simulink model "Predefined_with_GroundTruth_mod22vig1"  (R2022b)
settings: Solver=ode45  StartTime=0.0  StopTime=inf  MaxStep=0.01  RelTol=1e-3
PreLoadFcn:
  | old_index = 1;
model workspace (MAT data in the model file):
  firstWarning = 1
  originalScenarioChecksum = '114339432DE22364D47BB28FC96DC10C'
undefined symbols (not defined in the file or in its folder): Acceleration, ActorID, AngularVelocity, curvature, curvatureAhd, DefaultGear, DEND_B, DEND_S, DEND_T, direction, DiscIntNeverNeededParam, driving, gradbp, L, LF, LR, matlabshared, MAX_BRAKE, MAX_STEER, MAX_TORQUE, MCAR, MIN_BRAKE, MIN_STEER, MIN_TORQUE, NUMD_B, NUMD_S, NUMD_T, Pitch, Position, psi_o, R, Roll, RRdamp, SceneInfo, session, sigbuilder_block, STEER_RATIO, stopSign_ID, Tdead, thetaRefs, TL_ID, TrackWidth, Ts, ts, Vdead, Velocity, WB, X_o, xRef2, xRef2s, Y_o, Yaw, yRef2, yRef2s
libraries: mpcsigdimcheck_private x10, drivingscenarioandsensors x8, drivingvehiclecontroller x2, eeGeneralControl x2, slpidlib x2, simulink x2, trackingutilitieslib x2, mpclib x1, mpcadaslib x1, robotalgslib x1, simulink_extras x1, drivinglib x1
(part 2 of 3)

== system Predefined_with_GroundTruth_mod22vig1/Subsystem/Tracking ==
  Detections : Inport
  Camera : drivingscenarioandsensors/Vision Detection Generator  SensorIndex=1  DetectorOutput=Objects only  UpdateInterval=0.01  LaneUpdateInterval=0.1  SensorLocation=[1.9 0]  Height=1.1  Yaw=0  Pitch=1  Roll=0  BusNameSource=Auto  BusName=BusObjectDetections  BusName2Source=Auto  BusName2=BusLaneDetections  MaxNumDetectionsSource=Property  MaxNumDetections=10  MaxNumLanesSource=Property  MaxNumLanes=30  DetectionCoordinates=Ego Cartesian  SimulateUsing=Interpreted execution  MaxRange=150  BoundingBoxAccuracy=5  ProcessNoiseIntensity=5  MaxSpeed=100  MaxAllowedOcclusion=0.5  MinObjectImageSize=[2 2]  DetectionProbability=0.9  FalsePositivesPerImage=0.1  MinLaneImageSize=[20 3]  LaneBoundaryAccuracy=3  HasNoise=on  InitialSeedSource=Repeatable  InitialSeed=0  UsedSeed=0  ActorProfilesSource=From Scenario Reader block  ActorProfilesParameters=driving.internal.ActorProfilesParameters  ActorProfilesExpression=[struct('ActorID',1,'ClassID',1,'Length',4.7,'Width',1.8,'Height',1.4,'OriginOffset',[-1.35 0 0],'MeshVertices',[3.7 0.9 0.857439446366782;3.7 -0.9 0.857439446366782;3.7 -0.9 0.314878892733564;3.7 0.9 0.314878892733564;3.7 0.9 0.857439446366782;2.525 0.9 0.993079584775086;2.525 -0.9 0.993079584775086;3.7 -0.9 0.857439446366782;1.82 0.72 1.4;0.41 0.72 1.4;0.41 -0.72 1.4;1.82 -0.72 1.4;-0.295 0.9 0.993079584775086;-1 0.9 0.857439446366782;-1 -0.9 0.857439446366782;-0.295 -0.9 0.993079584775086;3.7 0.9 0.857439446366782;3.7 0.9 0.314878892733564;2.525 0.9 0.314878892733564;2.525 0.9 0.993079584775086;2.525 0.9 0.993079584775086;2.525 0.9 0.314878892733564;-0.295 0.9 0.314878892733564;-0.295 0.9 0.993079584775086;-0.295 0.9 0.993079584775086;-0.295 0.9 0.314878892733564;-1 0.9 0.355570934256055;-1 0.9 0.857439446366782;2.525 0.9 0.993079584775086;-0.295 0.9 0.993079584775086;0.41 0.72 1.4;1.82 0.72 1.4;3.7 -0.9 0.857439446366782;3.7 -0.9 0.314878892733564;2.525 -0.9 0.314878892733564;2.525 -0.9 0.993079584775086;2.525 -0.9 0.993079584775086;2.525 -0.9 0.314878892733564;-0.295 -0.9 0.314878892733564;-0.295 -0.9 0.993079584775086;-0.295 -0.9 0.993079584775086;-0.295 -0.9 0.314878892733564;-1 -0.9 0.355570934256055;-1 -0.9 0.857439446366782;2.525 -0.9 0.993079584775086;-0.295 -0.9 0.993079584775086;0.41 -0.72 1.4;1.82 -0.72 1.4;-0.295 0.9 0.993079584775086;-0.295 -0.9 0.993079584775086;0.41 -0.72 1.4;0.41 0.72 1.4;2.525 -0.9 0.993079584775086;1.82 -0.72 1.4;1.82 0.72 1.4;2.525 0.9 0.993079584775086;-1 0.9 0.857439446366782;-1 0.9 0.355570934256055;-1 -0.9 0.355570934256055;-1 -0.9 0.857439446366782;3.7 0.9 0.314878892733564;3.7 -0.9 0.314878892733564;-0.295 -0.9 0.314878892733564;-0.295 0.9 0.314878892733564;-0.295 0.9 0.314878892733564;-1 0.9 0.355570934256055;-1 -0.9 0.355570934256055;-0.295 -0.9 0.314878892733564;0 -0.63 0;0 -0.87 0;0.191030206995054 -0.63 0.0601365173421445;0.191030206995054 -0.87 0.0601365173421445;0.309093367795925 -0.63 0.217575963708927;0.309093367795925 -0.87 0.217575963708927;0.309093367795925 -0.63 0.412181821758201;0.309093367795925 -0.87 0.412181821758201;0.191030206995054 -0.63 0.569621268124983;0.191030206995054 -0.87 0.569621268124983;0 -0.63 0.629757785467128;0 -0.87 0.629757785467128;-0.191030206995054 -0.63 0.569621268124983;-0.191030206995054 -0.87 0.569621268124983;-0.309093367795925 -0.63 0.412181821758201;-0.309093367795925 -0.87 0.412181821758201;-0.309093367795925 -0.63 0.217575963708927;-0.309093367795925 -0.87 0.217575963708927;-0.191030206995054 -0.63 0.0601365173421445;-0.191030206995054 -0.87 0.0601365173421445;0 -0.63 0;0 -0.87 0;0 -0.63 0;0.191030206995054 -0.63 0.0601365173421445;0.309093367795925 -0.63 0.217575963708927;0.309093367795925 -0.63 0.412181821758201;0.191030206995054 -0.63 0.569621268124983;0 -0.63 0.629757785467128;-0.191030206995054 -0.63 0.569621268124983;-0.309093367795925 -0.63 0.412181821758201;-0.309093367795925 -0.63 0.217575963708927;-0.191030206995054 -0.63 0.0601365173421445;0 -0.87 0;0.191030206995054 -0.87 0.0601365173421445;0.309093367795925 -0.87 0.217575963708927;0.309093367795925 -0.87 0.412181821758201;0.191030206995054 -0.87 0.569621268124983;0 -0.87 0.629757785467128;-0.191030206995054 -0.87 0.569621268124983;-0.309093367795925 -0.87 0.412181821758201;-0.309093367795925 -0.87 0.217575963708927;-0.191030206995054 -0.87 0.0601365173421445;0 0.87 0;0 0.63 0;0.191030206995054 0.87 0.0601365173421445;0.191030206995054 0.63 0.0601365173421445;0.309093367795925 0.87 0.217575963708927;0.309093367795925 0.63 0.217575963708927;0.309093367795925 0.87 0.412181821758201;0.309093367795925 0.63 0.412181821758201;0.191030206995054 0.87 0.569621268124983;0.191030206995054 0.63 0.569621268124983;0 0.87 0.629757785467128;0 0.63 0.629757785467128;-0.191030206995054 0.87 0.569621268124983;-0.191030206995054 0.63 0.569621268124983;-0.309093367795925 0.87 0.412181821758201;-0.309093367795925 0.63 0.412181821758201;-0.309093367795925 0.87 0.217575963708927;-0.309093367795925 0.63 0.217575963708927;-0.191030206995054 0.87 0.0601365173421445;-0.191030206995054 0.63 0.0601365173421445;0 ...(+3718 chars)],'MeshFaces',[1 2 3;3 4 1;5 6 7;7 8 5;9 10 11;11 12 9;13 14 15;15 16 13;17 18 19;19 20 17;21 22 23;23 24 21;25 26 27;27 28 25;29 30 31;31 32 29;33 34 35;35 36 33;37 38 39;39 40 37;41 42 43;43 44 41;45 46 47;47 48 45;49 50 51;51 52 49;53 54 55;55 56 53;57 58 59;59 60 57;61 62 63;63 64 61;65 66 67;67 68 65;69 71 72;72 70 69;71 73 74;74 72 71;73 75 76;76 74 73;75 77 78;78 76 75;77 79 80;80 78 77;79 81 82;82 80 79;81 83 84;84 82 81;83 85 86;86 84 83;85 87 88;88 86 85;87 89 90;90 88 87;91 92 93;91 93 94;91 94 95;91 95 96;91 96 97;91 97 98;91 98 99;91 99 100;101 102 103;101 103 104;101 104 105;101 105 106;101 106 107;101 107 108;101 108 109;101 109 110;111 113 114;114 112 111;113 115 116;116 114 113;115 117 118;118 116 115;117 119 120;120 118 117;119 121 122;122 120 119;121 123 124;124 122 121;123 125 126;126 124 123;125 127 128;128 126 125;127 129 130;130 128 127;129 131 132;132 130 129;133 134 135;133 135 136;133 136 137;133 137 138;133 138 139;133 139 140;133 140 141;133 141 142;143 144 145;143 145 146;143 146 147;143 147 148;143 148 149;143 149 150;143 150 151;143 151 152;153 155 156;156 154 153;155 157 158;158 156 155;157 159 160;160 158 157;159 161 162;162 160 159;161 163 164;164 162 161;163 165 166;166 164 163;165 167 168;168 166 165;167 169 170;170 168 167;169 171 172;172 170 169;171 173 174;174 172 171;175 176 177;175 177 178;175 178 179;175 179 180;175 180 181;175 181 182;175 182 183;175 183 184;185 186 187;185 187 188;185 188 189;185 189 190;185 190 191;185 191 192;185 192 193;185 193 194;195 197 198;198 196 195;197 199 200;200 198 197;199 201 202;202 200 199;201 203 204;204 202 201;203 205 206;206 204 203;205 207 208;208 206 205;207 209 210;210 208 207;209 211 212;212 210 209;211 213 214;214 212 211;213 215 216;216 214 213;217 218 219;217 219 220;217 220 221;217 221 222;217 222 223;217 223 224;217 224 225;217 225 226;227 228 229;227 229 230;227 230 231;227 231 232;227 232 233;227 233 234;227 234 235;227 235 236],'RCSPattern',[10 10;10 10],'RCSAzimuthAngles',[-180 180],'RCSElevationAngles',[-90 90]); struct('ActorID',2,'ClassID',7,'Length',0.7,'Width',0.2,'Height',0.1,'OriginOffset',[0 0 0],'MeshVertices',[0.35 -0.1 0.1;0.35 0.1 0.1;-0.35 0.1 0.1;-0.35 -0.1 0.1;0.35 -0.1 0;0.35 0.1 0;-0.35 0.1 0;-0.35 -0.1 0],'MeshFaces',[6 2 1;1 5 6;8 4 3;3 7 8;6 7 3;3 2 6;5 1 4;4 8 5;4 1 2;2 3 4;7 6 5;5 8 7],'RCSPattern',[10 10;10 10],'RCSAzimuthAngles',[-180 180],'RCSElevationAngles',[-90 90])]  Intrinsics=driving.internal.cameraIntrinsics('FocalLength',[400 800],'PrincipalPoint',[320 240],'ImageSize',[480 640],'RadialDistortion',[0 0],'TangentialDistortion',[0 0],'Skew',0)
  Detection Concatenation : trackingutilitieslib/Detection Concatenation  NumInputs=2  BusNameSource=Property  BusName=Detections  SimulateUsing=Interpreted execution
  Multi-Object Tracker : drivinglib/Multi-Object Tracker  TrackerIndex=uint32( 0 )  FilterInitializationFcn=helperInitSimulinkDemoFilter  AssignmentThreshold=50  ConfirmationThreshold=[ 2, 3 ]  DeletionThreshold=[ 5, 5 ]  MaxNumTracks=20  MaxNumSensors=20  OOSMHandling=Neglect  StateParametersSimulink=struct  HasStateParametersInput=off  TimeInputSource=Auto  HasCostMatrixInput=off  HasDetectableTrackIDsInput=off  BusNameSource=Auto  BusName=BusMultiObjectTracker  TentativeTracksOutputPort=off  AllTracksOutputPort=off  SimulateUsing=Interpreted execution
  Radar Detection Generator : drivingscenarioandsensors/Radar Detection Generator  SensorIndex=2  UpdateInterval=0.01  SensorLocation=[ 1.5, 0 ]  Height=0.2  Yaw=0  Pitch=0  Roll=0  BusNameSource=Auto  BusName=BusRadarDetectionGenerator  MaxNumDetectionsSource=Property  MaxNumDetections=50  DetectionCoordinates=Ego Cartesian  SimulateUsing=Interpreted execution  AzimuthResolution=4  ElevationResolution=10  RangeResolution=2.5  RangeRateResolution=0.5  AzimuthBiasFraction=0.1  ElevationBiasFraction=0.1  RangeBiasFraction=0.05  RangeRateBiasFraction=0.05  FieldOfView=[ 60, 5 ]  MaxRange=150  RangeRateLimits=[ -100, 100 ]  DetectionProbability=0.9  FalseAlarmRate=1e-6  ReferenceRange=100  ReferenceRCS=0  HasElevation=off  HasRangeRate=on  HasNoise=on  HasFalseAlarms=on  HasOcclusion=on  InitialSeedSource=Repeatable  InitialSeed=0  UsedSeed=matlabshared.tracking.internal.SimulinkUtilities.seedManager(gcb)  ActorProfilesSource=Parameters  ActorProfilesParameters=driving.internal.ActorProfilesRadarParameters  ActorProfilesExpression=struct( 'ClassID', 0, 'Length', 4.7, 'Width', 1.8, 'Height', 1.4, 'OriginOffset', [ -1.35, 0, 0 ], 'RCSPattern', [ 10, 10; 10, 10 ], 'RCSAzimuthAngles', [ -180, 180 ], 'RCSElevationAngles', [ -90, 90 ] )
  Subsystem1 : Subsystem  Commented=on
  Confirmed_Tracks : Outport
  wires:
  Camera/1 -> Detection Concatenation/1  "Camera Detections"
  Radar Detection Generator/1 -> Detection Concatenation/2  "Lidar Detections"
  Detections/1 -> Radar Detection Generator/1, Camera/1
  Detection Concatenation/1 -> Multi-Object Tracker/1
  Multi-Object Tracker/1 -> Confirmed_Tracks/1

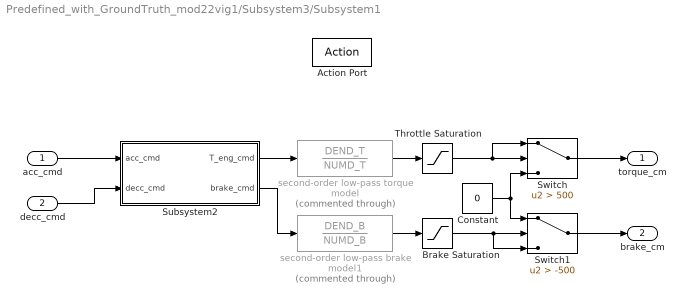
== system Predefined_with_GroundTruth_mod22vig1/Subsystem3/Subsystem1 ==
  acc_cmd : Inport
  decc_cmd : Inport  Port=2
  Action Port : ActionPort  ActionPortLabel=case [ 0 ]:
  Brake Saturation : Saturate  UpperLimit=MAX_BRAKE  LowerLimit=MIN_BRAKE
  Constant : Constant  Value=0
  Subsystem2 : Subsystem
  Switch : Switch  Criteria=u2 > Threshold  Threshold=500  SaturateOnIntegerOverflow=off  InputSameDT=off
  Switch1 : Switch  Criteria=u2 > Threshold  Threshold=-500  SaturateOnIntegerOverflow=off  InputSameDT=off
  Throttle Saturation : Saturate  UpperLimit=MAX_TORQUE  LowerLimit=MIN_TORQUE
  second-order low-pass brake model1 : DiscreteTransferFcn  Commented=through  Numerator=DEND_B  Denominator=NUMD_B  SampleTime=ts
  second-order low-pass torque model : DiscreteTransferFcn  Commented=through  Numerator=DEND_T  Denominator=NUMD_T  SampleTime=ts
  torque_cm : Outport
  brake_cm : Outport  Port=2
  wires:
  Subsystem2/1(T_eng_cmd) -> second-order low-pass torque model/1
  acc_cmd/1 -> Subsystem2/1(acc_cmd)
  second-order low-pass brake model1/1 -> Brake Saturation/1
  Subsystem2/2(brake_cmd) -> second-order low-pass brake model1/1
  decc_cmd/1 -> Subsystem2/2(decc_cmd)
  second-order low-pass torque model/1 -> Throttle Saturation/1
  Throttle Saturation/1 -> Switch/2, Switch/1
  Switch/1 -> torque_cm/1
  Brake Saturation/1 -> Switch1/2, Switch1/3
  Switch1/1 -> brake_cm/1
  Constant/1 -> Switch/3, Switch1/1

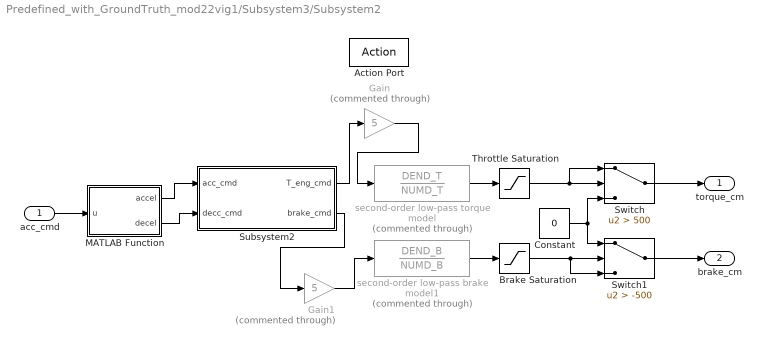
== system Predefined_with_GroundTruth_mod22vig1/Subsystem3/Subsystem2 ==
  acc_cmd : Inport
  Action Port : ActionPort  ActionPortLabel=case [ 1 ]:
  Brake Saturation : Saturate  UpperLimit=MAX_BRAKE  LowerLimit=MIN_BRAKE
  Constant : Constant  Value=0
  Gain : Gain  Commented=through  Gain=5
  Gain1 : Gain  Commented=through  Gain=5
  MATLAB Function : MATLAB Function  TreatAsAtomicUnit=on
  Subsystem2 : Subsystem
  Switch : Switch  Criteria=u2 > Threshold  Threshold=500  SaturateOnIntegerOverflow=off  InputSameDT=off
  Switch1 : Switch  Criteria=u2 > Threshold  Threshold=-500  SaturateOnIntegerOverflow=off  InputSameDT=off
  Throttle Saturation : Saturate  UpperLimit=MAX_TORQUE  LowerLimit=MIN_TORQUE
  second-order low-pass brake model1 : DiscreteTransferFcn  Commented=through  Numerator=DEND_B  Denominator=NUMD_B  SampleTime=ts
  second-order low-pass torque model : DiscreteTransferFcn  Commented=through  Numerator=DEND_T  Denominator=NUMD_T  SampleTime=ts
  torque_cm : Outport
  brake_cm : Outport  Port=2
  wires:
  second-order low-pass brake model1/1 -> Brake Saturation/1
  second-order low-pass torque model/1 -> Throttle Saturation/1
  Throttle Saturation/1 -> Switch/2, Switch/1
  Switch/1 -> torque_cm/1
  Brake Saturation/1 -> Switch1/2, Switch1/3
  Switch1/1 -> brake_cm/1
  Constant/1 -> Switch/3, Switch1/1
  acc_cmd/1 -> MATLAB Function/1(u)
  MATLAB Function/1(accel) -> Subsystem2/1(acc_cmd)
  MATLAB Function/2(decel) -> Subsystem2/2(decc_cmd)
  Subsystem2/1(T_eng_cmd) -> Gain/1
  Gain/1 -> second-order low-pass torque model/1
  Gain1/1 -> second-order low-pass brake model1/1
  Subsystem2/2(brake_cmd) -> Gain1/1

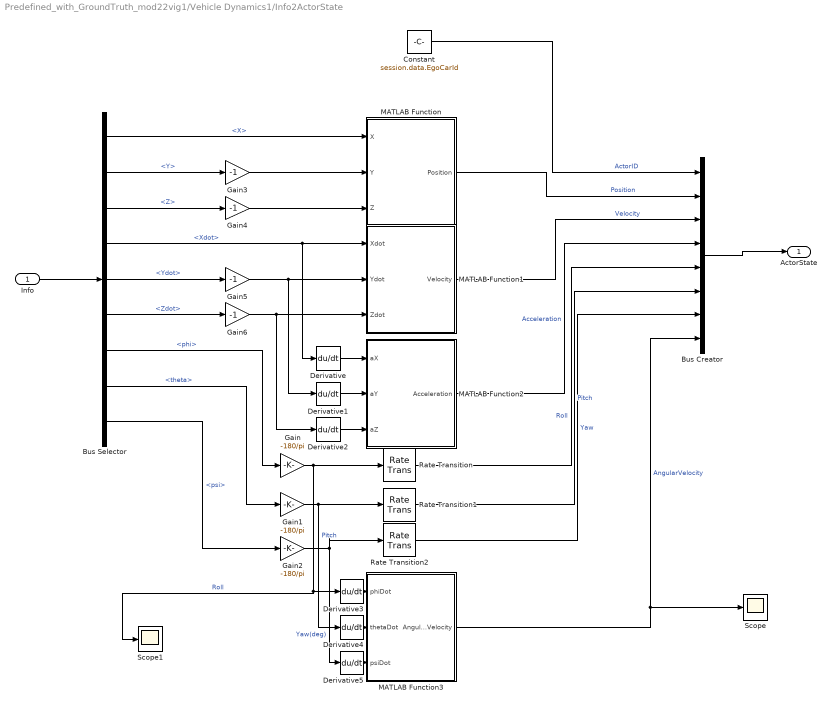
== system Predefined_with_GroundTruth_mod22vig1/Vehicle Dynamics1/Info2ActorState ==
  Info : Inport
  Bus Creator : BusCreator  Inputs=ActorID,Position,Velocity,Acceleration,Roll,Pitch,Yaw,AngularVelocity  OutDataTypeStr=Bus: BusActorState  NonVirtualBus=on
  Bus Selector : BusSelector  OutputSignals=InertFrm.Cg.Disp.X,InertFrm.Cg.Disp.Y,InertFrm.Cg.Disp.Z,InertFrm.Cg.Vel.Xdot,InertFrm.Cg.Vel.Ydot,InertFrm.Cg.Vel.Zdot,InertFrm.Cg.Ang.phi,InertFrm.Cg.Ang.theta,InertFrm.Cg.Ang.psi
  Constant : Constant  Value=session.data.EgoCarId  SampleTime=0.05
  Derivative{,1..5} (6 alike) : Derivative
  Gain : Gain  Gain=-180/pi
  Gain1 : Gain  Gain=-180/pi
  Gain2 : Gain  Gain=-180/pi
  Gain{3..6} (4 alike) : Gain  Gain=-1
  MATLAB Function : MATLAB Function  TreatAsAtomicUnit=on  SystemSampleTime=0.05
  MATLAB Function1 : MATLAB Function  TreatAsAtomicUnit=on  SystemSampleTime=0.05
  MATLAB Function2 : MATLAB Function  TreatAsAtomicUnit=on  SystemSampleTime=0.05
  MATLAB Function3 : MATLAB Function  TreatAsAtomicUnit=on  SystemSampleTime=0.05
  Rate Transition : RateTransition  OutPortSampleTime=0.05
  Rate Transition1 : RateTransition  OutPortSampleTime=0.05
  Rate Transition2 : RateTransition  OutPortSampleTime=0.05
  Scope : Scope
  Scope1 : Scope
  ActorState : Outport
  wires:
  Gain/1 -> Scope1/1, Derivative3/1, Rate Transition/1  "Roll"
  Derivative4/1 -> MATLAB Function3/2(thetaDot)
  Bus Selector/2 -> Gain3/1  "<Y>"
  Bus Selector/4 -> Derivative/1, MATLAB Function1/1(Xdot)  "<Xdot>"
  MATLAB Function1/1(Velocity) -> Bus Creator/3  "Velocity"
  MATLAB Function/1(Position) -> Bus Creator/2  "Position"
  Derivative1/1 -> MATLAB Function2/2(aY)
  Bus Selector/5 -> Gain5/1  "<Ydot>"
  Bus Selector/1 -> MATLAB Function/1(X)  "<X>"
  Bus Selector/9 -> Gain2/1  "<psi>"
  Gain2/1 -> Rate Transition2/1, Derivative5/1  "Yaw(deg)"
  Derivative5/1 -> MATLAB Function3/3(psiDot)
  Bus Selector/7 -> Gain/1  "<phi>"
  MATLAB Function2/1(Acceleration) -> Bus Creator/4  "Acceleration"
  Derivative3/1 -> MATLAB Function3/1(phiDot)
  Gain1/1 -> Derivative4/1, Rate Transition1/1  "Pitch"
  Bus Selector/6 -> Gain6/1  "<Zdot>"
  Bus Selector/8 -> Gain1/1  "<theta>"
  MATLAB Function3/1(AngularVelocity) -> Bus Creator/8, Scope/1  "AngularVelocity"
  Bus Selector/3 -> Gain4/1  "<Z>"
  Derivative2/1 -> MATLAB Function2/3(aZ)
  Derivative/1 -> MATLAB Function2/1(aX)
  Info/1 -> Bus Selector/1
  Constant/1 -> Bus Creator/1  "ActorID"
  Bus Creator/1 -> ActorState/1
  Rate Transition/1 -> Bus Creator/5  "Roll"
  Rate Transition1/1 -> Bus Creator/6  "Pitch"
  Rate Transition2/1 -> Bus Creator/7  "Yaw"
  Gain3/1 -> MATLAB Function/2(Y)
  Gain4/1 -> MATLAB Function/3(Z)
  Gain5/1 -> Derivative1/1, MATLAB Function1/2(Ydot)
  Gain6/1 -> Derivative2/1, MATLAB Function1/3(Zdot)

== system Predefined_with_GroundTruth_mod22vig1/Vehicle Dynamics1/Subsystem ==
  Gain : Gain  Gain=MAX_TORQUE*0.1
  Gain1 : Gain  Gain=MIN_BRAKE*0.06
  Gain2 : Gain  Gain=MAX_STEER/4.5
  Signal Builder : Subsystem  Tag=STV Subsys  LoadFcn=sigbuilder_block('load');  StartFcn=sigbuilder_block('start');  StopFcn=sigbuilder_block('stop');  ClipboardFcn=sigbuilder_block('clipboard');  mask(Sigbuilder block){tuvar=[0:10]}
      mask help: Simulink:masks:SigbuilderBlock_MD
      mask init:
      | if ~strcmp(get_param(bdroot(gcbh),'SimulationStatus'),'stopped') tuvar = sigbuilder_block('maskInit'); end
      settings: CopyFcn=sigbuilder_block('copy');  DeleteFcn=sigbuilder_block('delete');  ModelCloseFcn=sigbuilder_block('modelClose');  PreSaveFcn=sigbuilder_block('preSave');  PauseFcn=sigbuilder_block('pause');  ContinueFcn=sigbuilder_block('continue');  NameChangeFcn=sigbuilder_block('namechange');  OpenFcn=sigbuilder_block('open',[0 30 960 455.5 ]);  CloseFcn=sigbuilder_block('close');
      mask Display: plot(0, 0, 100, 100,[2, 2, 32, 32, 2], [68, 8, 8, 68, 68],[32, 2], [38, 38], [32, 19, 2],[53, 60, 44], [32, 17, 17, 2],[16, 16, 31, 31]);txt = getActiveGroup(gcbh);text(2, 100, txt,'verticalAlignment', 'top');
  torque_cmd (Nm) : Outport
  brake_cmd (Nm) : Outport  Port=2
  steer_cmd (deg) : Outport  Port=3
  wires:
  Gain2/1 -> steer_cmd (deg)/1  "steer_cmd (deg)"
  Signal Builder/1(Normalized Torque) -> Gain/1
  Signal Builder/2(Normalized Brake) -> Gain1/1
  Signal Builder/3(Normalized Steer) -> Gain2/1  "steer_cmd (deg)"
  Gain1/1 -> brake_cmd (Nm)/1  "brake_cmd (Nm)"
  Gain/1 -> torque_cmd (Nm)/1  "torque_cmd (Nm)"

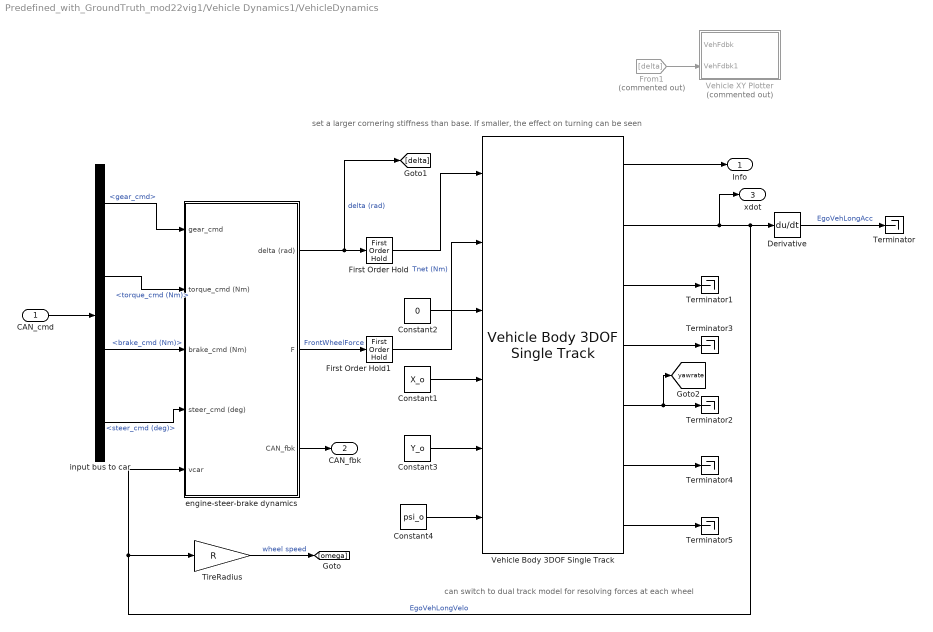
== system Predefined_with_GroundTruth_mod22vig1/Vehicle Dynamics1/VehicleDynamics ==
  note: set a larger cornering stiffness than base. If smaller, the effect on turning can be seen
  note: can switch to dual track model for resolving forces at each wheel
  CAN_cmd : Inport
  Constant1 : Constant  Value=X_o
  Constant2 : Constant  Value=0
  Constant3 : Constant  Value=Y_o
  Constant4 : Constant  Value=psi_o
  Derivative : Derivative
  First Order Hold : FirstOrderHold  ErrorTolerance=inf
  First Order Hold1 : FirstOrderHold  ErrorTolerance=inf
  From1 : From  Commented=on  GotoTag=delta
  Terminator{,1..5} (6 alike) : Terminator
  TireRadius : Gain  Gain=R
  Vehicle Body 3DOF Single Track : autolibshared/Vehicle Body 3DOF Single Track  trackMode=Single (bicycle)  inputMode=External longitudinal forces  frontSteerMode=on  rearSteerMode=off  windMode=off  muMode=off  extFMode=off  extMMode=off  htchFMode=off  htchMMode=off  extXo=on  extpsio=on  extxdoto=off  extro=off  extYo=on  extTamb=off  extydoto=off  aMode=2  NF=2  NR=2  m=MCAR  a=LF  b=LR  h=0.35  dh=1  hh=0.2  X_o=InitPosition(1)  xdot_o=InitSpeed  CalphaMode=off  sigmaMode=on  d=0  hl=0  w=[1.4,1.4]  Cy_f=12e3*100  Cy_r=11e3*100  sigma_f=.1  sigma_r=.1  alpha_f_brk=[-.1 .1]  Cy_f_data=[-9e3 9e3]  alpha_r_brk=[-.1 .1]  Cy_r_data=[-9e3 9e3]  Y_o=-InitPosition(2)  ydot_o=0  Izz=2050  psi_o=-InitYaw/180*pi  r_o=0  Af=2  Cd=.3  Cl=.1  Cpm=.1  beta_w=[0:0.01:0.3]  Cs=[0:0.03:0.9]  Cym=[0:0.01:0.3]  Pabs=101325  Tair=273  g=9.81  mu=1  xdot_tol=.01  Fznom=5000  Fxtire_sat=7e4  Fytire_sat=7e4  longOff=0  latOff=0  vertOff=0  wrapAng=off
  Vehicle XY Plotter : Subsystem  Commented=on  mask(Vehicle XY Plotter){a=LF, b=LR, w=TrackWidth, bufferSize=1024, pltDT=.1}
      mask prompts: a "Distance to front axle from CG, a [m]:"; b "Distance to rear axle from CG, b [m]:"; w "Track width, w [m]:"; bufferSize "Path buffer sampe size, bufferSize []:"; pltDT "Plot update rate, pltDT [s]:"
      mask help: This block will display a MATLAB figure which indicates the vehicle path, current position and heading velocity.
      mask TypeOptions a: Vehicle XY Plotter/a
      mask TypeOptions b: Vehicle XY Plotter/b
      mask TypeOptions w: Vehicle XY Plotter/w
      mask TypeOptions bufferSize: Vehicle XY Plotter/bufferSize
  engine-steer-brake dynamics : Subsystem
  input bus to car : BusSelector  OutputSignals=gear_cmd,torque_cmd (Nm),brake_cmd (Nm),steer_cmd (deg)
  Info : Outport
  CAN_fbk : Outport  Port=2  VectorParamsAs1DForOutWhenUnconnected=off
  xdot : Outport  Port=3
  tag scope: yawrate=global
  wires:
  TireRadius/1 -> [omega]  "wheel speed"
  Vehicle Body 3DOF Single Track/1 -> Info/1
  From1/1 -> Vehicle XY Plotter/2(VehFdbk1)
  input bus to car/1 -> engine-steer-brake dynamics/1(gear_cmd)  "<gear_cmd>"
  input bus to car/3 -> engine-steer-brake dynamics/3(brake_cmd (Nm))  "<brake_cmd (Nm)>"
  engine-steer-brake dynamics/1(delta (rad)) -> [delta], First Order Hold/1  "delta (rad)"
  input bus to car/2 -> engine-steer-brake dynamics/2(torque_cmd (Nm))  "<torque_cmd (Nm)>"
  input bus to car/4 -> engine-steer-brake dynamics/4(steer_cmd (deg))  "<steer_cmd (deg)>"
  engine-steer-brake dynamics/3(CAN_fbk) -> CAN_fbk/1
  CAN_cmd/1 -> input bus to car/1
  Constant2/1 -> Vehicle Body 3DOF Single Track/3
  engine-steer-brake dynamics/2(F) -> First Order Hold1/1  "FrontWheelForce"
  First Order Hold/1 -> Vehicle Body 3DOF Single Track/1
  Vehicle Body 3DOF Single Track/2 -> xdot/1, engine-steer-brake dynamics/5(vcar), TireRadius/1, Derivative/1  "EgoVehLongVelo"
  Vehicle Body 3DOF Single Track/3 -> Terminator1/1
  Vehicle Body 3DOF Single Track/4 -> Terminator3/1
  Vehicle Body 3DOF Single Track/5 -> [yawrate], Terminator2/1
  Vehicle Body 3DOF Single Track/6 -> Terminator4/1
  Vehicle Body 3DOF Single Track/7 -> Terminator5/1
  Derivative/1 -> Terminator/1  "EgoVehLongAcc"
  First Order Hold1/1 -> Vehicle Body 3DOF Single Track/2  "Tnet (Nm)"
  Constant1/1 -> Vehicle Body 3DOF Single Track/4
  Constant3/1 -> Vehicle Body 3DOF Single Track/5
  Constant4/1 -> Vehicle Body 3DOF Single Track/6

== system Predefined_with_GroundTruth_mod22vig1/Reference Data/Theta/thetaBlocks ==
  note: theta calculated from Simulink blocks
  y : Inport
  x : Inport  Port=2
  dis : Inport  Port=3
  Atan2 : Trigonometry  Operator=atan2  ApproximationMethod=CORDIC
  Difference : simulink/Discrete/Difference  ICPrevInput=0.0  OutMin=[]  OutMax=[]  OutDataType=fixdt(1, 16)  OutScaling=2^-10  DoSatur=off
  Difference1 : simulink/Discrete/Difference  ICPrevInput=0.0  OutMin=[]  OutMax=[]  OutDataType=fixdt(1, 16)  OutScaling=2^-10  DoSatur=off
  IC : InitialCondition  Value=psi_o
  Radians to Degrees : simulink_extras/Transformations/Radians to Degrees
  Terminator : Terminator
  theta : Outport
  wires:
  IC/1 -> Radians to Degrees/1
  Atan2/1 -> IC/1
  dis/1 -> Terminator/1
  x/1 -> Difference1/1
  y/1 -> Difference/1
  Radians to Degrees/1 -> theta/1
  Difference/1 -> Atan2/1
  Difference1/1 -> Atan2/2

== system Predefined_with_GroundTruth_mod22vig1/Reference Data/Theta/thetaLt ==
  note: Check out the script "setUpModel" to understand how we have calculated theta
  note: theta based on lookup table
  y : Inport
  x : Inport  Port=2
  dis : Inport  Port=3
  Terminator : Terminator
  Terminator1 : Terminator
  Theta Ref : Lookup_n-D  NumberOfTableDimensions=1  BreakpointsForDimension1=gradbp  Table=thetaRefs  InternalRulePriority=Speed  RndMeth=Simplest
  theta : Outport
  wires:
  Theta Ref/1 -> theta/1
  dis/1 -> Theta Ref/1
  x/1 -> Terminator1/1
  y/1 -> Terminator/1

== system Predefined_with_GroundTruth_mod22vig1/Subsystem/Tracking/Subsystem1 ==
  In2 : Inport
  EgoV : Inport  Port=2
  Camera : drivingscenarioandsensors/Vision Detection Generator  SensorIndex=1  DetectorOutput=Objects only  UpdateInterval=0.1  LaneUpdateInterval=0.1  SensorLocation=[1.9 0]  Height=1.1  Yaw=0  Pitch=1  Roll=0  BusNameSource=Auto  BusName=BusObjectDetections  BusName2Source=Auto  BusName2=BusLaneDetections  MaxNumDetectionsSource=Property  MaxNumDetections=10  MaxNumLanesSource=Property  MaxNumLanes=30  DetectionCoordinates=Ego Cartesian  SimulateUsing=Interpreted execution  MaxRange=150  BoundingBoxAccuracy=5  ProcessNoiseIntensity=5  MaxSpeed=100  MaxAllowedOcclusion=0.5  MinObjectImageSize=[5 5]  DetectionProbability=0.9  FalsePositivesPerImage=0.1  MinLaneImageSize=[20 3]  LaneBoundaryAccuracy=3  HasNoise=on  InitialSeedSource=Repeatable  InitialSeed=0  UsedSeed=0  ActorProfilesSource=From Scenario Reader block  ActorProfilesParameters=driving.internal.ActorProfilesParameters  ActorProfilesExpression=[struct('ActorID',1,'ClassID',1,'Length',4.7,'Width',1.8,'Height',1.4,'OriginOffset',[-1.35 0 0],'MeshVertices',[3.7 0.9 0.857439446366782;3.7 -0.9 0.857439446366782;3.7 -0.9 0.314878892733564;3.7 0.9 0.314878892733564;3.7 0.9 0.857439446366782;2.525 0.9 0.993079584775086;2.525 -0.9 0.993079584775086;3.7 -0.9 0.857439446366782;1.82 0.72 1.4;0.41 0.72 1.4;0.41 -0.72 1.4;1.82 -0.72 1.4;-0.295 0.9 0.993079584775086;-1 0.9 0.857439446366782;-1 -0.9 0.857439446366782;-0.295 -0.9 0.993079584775086;3.7 0.9 0.857439446366782;3.7 0.9 0.314878892733564;2.525 0.9 0.314878892733564;2.525 0.9 0.993079584775086;2.525 0.9 0.993079584775086;2.525 0.9 0.314878892733564;-0.295 0.9 0.314878892733564;-0.295 0.9 0.993079584775086;-0.295 0.9 0.993079584775086;-0.295 0.9 0.314878892733564;-1 0.9 0.355570934256055;-1 0.9 0.857439446366782;2.525 0.9 0.993079584775086;-0.295 0.9 0.993079584775086;0.41 0.72 1.4;1.82 0.72 1.4;3.7 -0.9 0.857439446366782;3.7 -0.9 0.314878892733564;2.525 -0.9 0.314878892733564;2.525 -0.9 0.993079584775086;2.525 -0.9 0.993079584775086;2.525 -0.9 0.314878892733564;-0.295 -0.9 0.314878892733564;-0.295 -0.9 0.993079584775086;-0.295 -0.9 0.993079584775086;-0.295 -0.9 0.314878892733564;-1 -0.9 0.355570934256055;-1 -0.9 0.857439446366782;2.525 -0.9 0.993079584775086;-0.295 -0.9 0.993079584775086;0.41 -0.72 1.4;1.82 -0.72 1.4;-0.295 0.9 0.993079584775086;-0.295 -0.9 0.993079584775086;0.41 -0.72 1.4;0.41 0.72 1.4;2.525 -0.9 0.993079584775086;1.82 -0.72 1.4;1.82 0.72 1.4;2.525 0.9 0.993079584775086;-1 0.9 0.857439446366782;-1 0.9 0.355570934256055;-1 -0.9 0.355570934256055;-1 -0.9 0.857439446366782;3.7 0.9 0.314878892733564;3.7 -0.9 0.314878892733564;-0.295 -0.9 0.314878892733564;-0.295 0.9 0.314878892733564;-0.295 0.9 0.314878892733564;-1 0.9 0.355570934256055;-1 -0.9 0.355570934256055;-0.295 -0.9 0.314878892733564;0 -0.63 0;0 -0.87 0;0.191030206995054 -0.63 0.0601365173421445;0.191030206995054 -0.87 0.0601365173421445;0.309093367795925 -0.63 0.217575963708927;0.309093367795925 -0.87 0.217575963708927;0.309093367795925 -0.63 0.412181821758201;0.309093367795925 -0.87 0.412181821758201;0.191030206995054 -0.63 0.569621268124983;0.191030206995054 -0.87 0.569621268124983;0 -0.63 0.629757785467128;0 -0.87 0.629757785467128;-0.191030206995054 -0.63 0.569621268124983;-0.191030206995054 -0.87 0.569621268124983;-0.309093367795925 -0.63 0.412181821758201;-0.309093367795925 -0.87 0.412181821758201;-0.309093367795925 -0.63 0.217575963708927;-0.309093367795925 -0.87 0.217575963708927;-0.191030206995054 -0.63 0.0601365173421445;-0.191030206995054 -0.87 0.0601365173421445;0 -0.63 0;0 -0.87 0;0 -0.63 0;0.191030206995054 -0.63 0.0601365173421445;0.309093367795925 -0.63 0.217575963708927;0.309093367795925 -0.63 0.412181821758201;0.191030206995054 -0.63 0.569621268124983;0 -0.63 0.629757785467128;-0.191030206995054 -0.63 0.569621268124983;-0.309093367795925 -0.63 0.412181821758201;-0.309093367795925 -0.63 0.217575963708927;-0.191030206995054 -0.63 0.0601365173421445;0 -0.87 0;0.191030206995054 -0.87 0.0601365173421445;0.309093367795925 -0.87 0.217575963708927;0.309093367795925 -0.87 0.412181821758201;0.191030206995054 -0.87 0.569621268124983;0 -0.87 0.629757785467128;-0.191030206995054 -0.87 0.569621268124983;-0.309093367795925 -0.87 0.412181821758201;-0.309093367795925 -0.87 0.217575963708927;-0.191030206995054 -0.87 0.0601365173421445;0 0.87 0;0 0.63 0;0.191030206995054 0.87 0.0601365173421445;0.191030206995054 0.63 0.0601365173421445;0.309093367795925 0.87 0.217575963708927;0.309093367795925 0.63 0.217575963708927;0.309093367795925 0.87 0.412181821758201;0.309093367795925 0.63 0.412181821758201;0.191030206995054 0.87 0.569621268124983;0.191030206995054 0.63 0.569621268124983;0 0.87 0.629757785467128;0 0.63 0.629757785467128;-0.191030206995054 0.87 0.569621268124983;-0.191030206995054 0.63 0.569621268124983;-0.309093367795925 0.87 0.412181821758201;-0.309093367795925 0.63 0.412181821758201;-0.309093367795925 0.87 0.217575963708927;-0.309093367795925 0.63 0.217575963708927;-0.191030206995054 0.87 0.0601365173421445;-0.191030206995054 0.63 0.0601365173421445;0 ...(+3718 chars)],'MeshFaces',[1 2 3;3 4 1;5 6 7;7 8 5;9 10 11;11 12 9;13 14 15;15 16 13;17 18 19;19 20 17;21 22 23;23 24 21;25 26 27;27 28 25;29 30 31;31 32 29;33 34 35;35 36 33;37 38 39;39 40 37;41 42 43;43 44 41;45 46 47;47 48 45;49 50 51;51 52 49;53 54 55;55 56 53;57 58 59;59 60 57;61 62 63;63 64 61;65 66 67;67 68 65;69 71 72;72 70 69;71 73 74;74 72 71;73 75 76;76 74 73;75 77 78;78 76 75;77 79 80;80 78 77;79 81 82;82 80 79;81 83 84;84 82 81;83 85 86;86 84 83;85 87 88;88 86 85;87 89 90;90 88 87;91 92 93;91 93 94;91 94 95;91 95 96;91 96 97;91 97 98;91 98 99;91 99 100;101 102 103;101 103 104;101 104 105;101 105 106;101 106 107;101 107 108;101 108 109;101 109 110;111 113 114;114 112 111;113 115 116;116 114 113;115 117 118;118 116 115;117 119 120;120 118 117;119 121 122;122 120 119;121 123 124;124 122 121;123 125 126;126 124 123;125 127 128;128 126 125;127 129 130;130 128 127;129 131 132;132 130 129;133 134 135;133 135 136;133 136 137;133 137 138;133 138 139;133 139 140;133 140 141;133 141 142;143 144 145;143 145 146;143 146 147;143 147 148;143 148 149;143 149 150;143 150 151;143 151 152;153 155 156;156 154 153;155 157 158;158 156 155;157 159 160;160 158 157;159 161 162;162 160 159;161 163 164;164 162 161;163 165 166;166 164 163;165 167 168;168 166 165;167 169 170;170 168 167;169 171 172;172 170 169;171 173 174;174 172 171;175 176 177;175 177 178;175 178 179;175 179 180;175 180 181;175 181 182;175 182 183;175 183 184;185 186 187;185 187 188;185 188 189;185 189 190;185 190 191;185 191 192;185 192 193;185 193 194;195 197 198;198 196 195;197 199 200;200 198 197;199 201 202;202 200 199;201 203 204;204 202 201;203 205 206;206 204 203;205 207 208;208 206 205;207 209 210;210 208 207;209 211 212;212 210 209;211 213 214;214 212 211;213 215 216;216 214 213;217 218 219;217 219 220;217 220 221;217 221 222;217 222 223;217 223 224;217 224 225;217 225 226;227 228 229;227 229 230;227 230 231;227 231 232;227 232 233;227 233 234;227 234 235;227 235 236],'RCSPattern',[10 10;10 10],'RCSAzimuthAngles',[-180 180],'RCSElevationAngles',[-90 90]); struct('ActorID',2,'ClassID',7,'Length',0.7,'Width',0.2,'Height',0.1,'OriginOffset',[0 0 0],'MeshVertices',[0.35 -0.1 0.1;0.35 0.1 0.1;-0.35 0.1 0.1;-0.35 -0.1 0.1;0.35 -0.1 0;0.35 0.1 0;-0.35 0.1 0;-0.35 -0.1 0],'MeshFaces',[6 2 1;1 5 6;8 4 3;3 7 8;6 7 3;3 2 6;5 1 4;4 8 5;4 1 2;2 3 4;7 6 5;5 8 7],'RCSPattern',[10 10;10 10],'RCSAzimuthAngles',[-180 180],'RCSElevationAngles',[-90 90])]  Intrinsics=driving.internal.cameraIntrinsics('FocalLength',[800 800],'PrincipalPoint',[320 240],'ImageSize',[480 640],'RadialDistortion',[0 0],'TangentialDistortion',[0 0],'Skew',0)
  Detection Concatenation : trackingutilitieslib/Detection Concatenation  NumInputs=3  BusNameSource=Auto  BusName=BusDetectionConcatenation  SimulateUsing=Interpreted execution
  Lidar Point Cloud Generator : drivingscenarioandsensors/Lidar Point Cloud Generator  SensorIndex=2  UpdateInterval=0.1  SensorLocation=[1.5 0]  Height=1.6  Yaw=0  Pitch=0  Roll=0  DetectionCoordinates=Ego Cartesian  HasEgoVehicle=on  EgoVehicleActorID=1  HasRoadsInputPort=on  ActorProfilesSource=From Scenario Reader block  ActorProfilesVariableName=actor_profiles  MaxRange=120  RangeAccuracy=0.002  AzimuthResolution=0.16  ElevationResolution=1.25  AzimuthLimits=[-60 60]  ElevationLimits=[ -20, 20 ]  HasNoise=on
  Lidar Point Cloud Generator1 : drivingscenarioandsensors/Lidar Point Cloud Generator  SensorIndex=3  UpdateInterval=0.1  SensorLocation=[1.5 0]  Height=1.6  Yaw=0  Pitch=0  Roll=0  DetectionCoordinates=Ego Cartesian  HasEgoVehicle=on  EgoVehicleActorID=1  HasRoadsInputPort=on  ActorProfilesSource=From Scenario Reader block  ActorProfilesVariableName=actor_profiles  MaxRange=120  RangeAccuracy=0.002  AzimuthResolution=0.16  ElevationResolution=1.25  AzimuthLimits=[60 180]  ElevationLimits=[ -20, 20 ]  HasNoise=on
  Lidar Point Cloud Generator2 : drivingscenarioandsensors/Lidar Point Cloud Generator  SensorIndex=4  UpdateInterval=0.1  SensorLocation=[1.5 0]  Height=1.6  Yaw=0  Pitch=0  Roll=0  DetectionCoordinates=Ego Cartesian  HasEgoVehicle=on  EgoVehicleActorID=1  HasRoadsInputPort=on  ActorProfilesSource=From Scenario Reader block  ActorProfilesVariableName=actor_profiles  MaxRange=120  RangeAccuracy=0.002  AzimuthResolution=0.16  ElevationResolution=1.25  AzimuthLimits=[-180 -60]  ElevationLimits=[ -20, 20 ]  HasNoise=on
  Camera Detections : Outport
  Radar detections : Outport  Port=2
  wires:
  EgoV/1 -> Lidar Point Cloud Generator1/2, Lidar Point Cloud Generator/2, Lidar Point Cloud Generator2/2
  Lidar Point Cloud Generator1/1 -> Detection Concatenation/2  "Lidar Detections"
  Lidar Point Cloud Generator2/1 -> Detection Concatenation/3  "Lidar Detections"
  Detection Concatenation/1 -> Radar detections/1
  Camera/1 -> Camera Detections/1  "Camera Detections"
  In2/1 -> Camera/1, Lidar Point Cloud Generator/1, Lidar Point Cloud Generator1/1, Lidar Point Cloud Generator2/1
  Lidar Point Cloud Generator/1 -> Detection Concatenation/1  "Lidar Detections"

== system Predefined_with_GroundTruth_mod22vig1/Subsystem3/Subsystem1/Subsystem2 ==
  acc_cmd : Inport
  decc_cmd : Inport  Port=2
  Subsystem : Subsystem
  Subsystem1 : Subsystem
  T_eng_cmd : Outport
  brake_cmd : Outport  Port=2
  wires:
  acc_cmd/1 -> Subsystem/1(acc_cmd)
  Subsystem/1(T_eng_cmd) -> T_eng_cmd/1
  decc_cmd/1 -> Subsystem1/1(decc_cmd)
  Subsystem1/1(T_brake_cmd) -> brake_cmd/1

== system Predefined_with_GroundTruth_mod22vig1/Subsystem3/Subsystem2/Subsystem2 ==
  acc_cmd : Inport
  decc_cmd : Inport  Port=2
  Subsystem : Subsystem
  Subsystem1 : Subsystem
  T_eng_cmd : Outport
  brake_cmd : Outport  Port=2
  wires:
  acc_cmd/1 -> Subsystem/1(acc_cmd)
  Subsystem/1(T_eng_cmd) -> T_eng_cmd/1
  decc_cmd/1 -> Subsystem1/1(decc_cmd)
  Subsystem1/1(T_brake_cmd) -> brake_cmd/1

== system Predefined_with_GroundTruth_mod22vig1/Vehicle Dynamics1/Subsystem/Signal Builder ==
  Demux : Demux  Tag=STV Demux  Outputs=3
      settings: DisplayOption=none
  FromWs : FromWorkspace  Tag=STV FromWs  VariableName=tuvar
      SigBuilderData=|
      | common.afterFinalStr = 'Extrapolate'
      | common.sampleTime = 0
      | dataSet.timeRange = [0 3.5]
      | dataSet.name = 'DriveAndTurn'
      | sbobj.Groups.Name = 'DriveAndTurn'
      | sbobj.Groups.Signals(1).Name = 'Normalized Torque'
      | sbobj.Groups.Signals(1).XData = [0 1 1 2 2 3.5]
      | sbobj.Groups.Signals(1).YData = [1 1 0 0 1 1]
      | sbobj.Groups.Signals(2).Name = 'Normalized Brake'
      | sbobj.Groups.Signals(2).XData = [0 1 1 2 2 3.5]
      | sbobj.Groups.Signals(2).YData = [0 0 1 1 0 0]
      | sbobj.Groups.Signals(3).Name = 'Normalized Steer'
      | sbobj.Groups.Signals(3).XData = [0 0.5 0.6 1.02 1.02 2 2.5 3 3.5]
      | sbobj.Groups.Signals(3).YData = [-0.02 -0.02 -0.02 -0.3 -1.02 -0.92 -0.34 0.14 0.22]
      | sbobj.Groups.TimeRange = [0 3.5]
  Normalized Torque : Outport  Tag=STV Outport
  Normalized Brake : Outport  Tag=STV Outport  Port=2
  Normalized Steer : Outport  Tag=STV Outport  Port=3
  wires:
  FromWs/1 -> Demux/1
  Demux/1 -> Normalized Torque/1
  Demux/2 -> Normalized Brake/1
  Demux/3 -> Normalized Steer/1

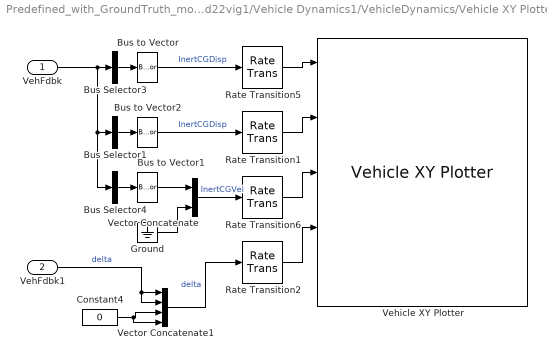
== system Predefined_with_GroundTruth_mod22vig1/Vehicle Dynamics1/VehicleDynamics/Vehicle XY Plotter ==
  VehFdbk : Inport
  VehFdbk1 : Inport  Port=2
  Bus Selector1 : BusSelector  OutputSignals=InertFrm.Cg.Ang.phi,InertFrm.Cg.Ang.theta,InertFrm.Cg.Ang.psi  OutputAsBus=on
  Bus Selector3 : BusSelector  OutputSignals=InertFrm.Geom.Disp.X,InertFrm.Geom.Disp.Y,InertFrm.Geom.Disp.Z  OutputAsBus=on
  Bus Selector4 : BusSelector  OutputSignals=InertFrm.Cg.Vel.Xdot,InertFrm.Cg.Vel.Ydot  OutputAsBus=on
  Bus to Vector : BusToVector
  Bus to Vector1 : BusToVector
  Bus to Vector2 : BusToVector
  Constant4 : Constant  Value=0
  Ground : Ground
  Rate Transition{1..2,5..6} (4 alike) : RateTransition  OutPortSampleTime=pltDT
  Vector Concatenate : Concatenate
  Vector Concatenate1 : Concatenate  NumInputs=4
  Vehicle XY Plotter : vehdynlibviscommon/Vehicle XY Plotter  w=w  a=a  b=b  figBorder=2000  bufferSize=bufferSize  extStats=off  extTireF=off
  wires:
  Bus to Vector2/1 -> Rate Transition1/1  "InertCGDisp"
  Rate Transition5/1 -> Vehicle XY Plotter/1
  Bus Selector4/1 -> Bus to Vector1/1
  Rate Transition1/1 -> Vehicle XY Plotter/2
  Rate Transition6/1 -> Vehicle XY Plotter/3
  Vector Concatenate/1 -> Rate Transition6/1  "InertCGVel"
  Bus Selector1/1 -> Bus to Vector2/1
  Bus to Vector/1 -> Rate Transition5/1  "InertCGDisp"
  Bus Selector3/1 -> Bus to Vector/1
  Bus to Vector1/1 -> Vector Concatenate/1
  Ground/1 -> Vector Concatenate/2
  VehFdbk/1 -> Bus Selector1/1, Bus Selector4/1, Bus Selector3/1
  Rate Transition2/1 -> Vehicle XY Plotter/4
  Constant4/1 -> Vector Concatenate1/4, Vector Concatenate1/3
  VehFdbk1/1 -> Vector Concatenate1/2, Vector Concatenate1/1  "delta"
  Vector Concatenate1/1 -> Rate Transition2/1  "delta"
